simulink subsystem "Encoder"  (R2024b)
settings: Solver=VariableStepAuto  StartTime=0.0  StopTime=10.0  RelTol=1e-3
undefined symbols (not defined in the file or in its folder): sens, Ts
settings Model: Creator=Riccardo Grosso  LastModifiedBy=Federico Bergami

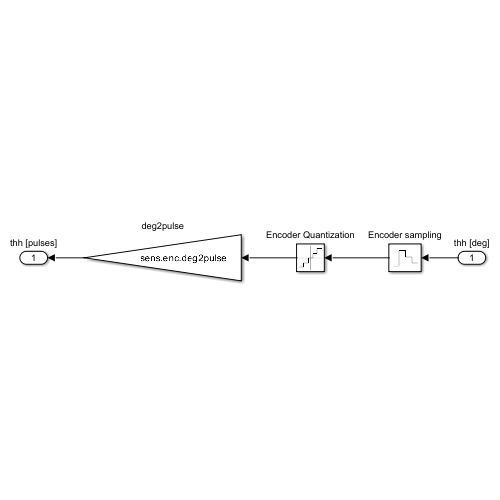
[thumbnail: Simulink's stored preview of the top-level diagram]
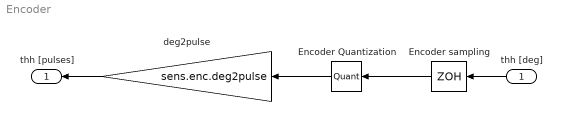
== system Encoder ==
  thh [deg] : Inport
  Encoder Quantization : Quantizer  QuantizationInterval=sens.enc.pulse2deg
  Encoder sampling : ZeroOrderHold  SampleTime=Ts
  deg2pulse : Gain  Gain=sens.enc.deg2pulse
  thh [pulses] : Outport
  wires:
  Encoder sampling/1 -> Encoder Quantization/1
  Encoder Quantization/1 -> deg2pulse/1
  thh [deg]/1 -> Encoder sampling/1
  deg2pulse/1 -> thh [pulses]/1
